simulink model "lte4g"  (R2020b)
settings: Solver=ode45  StartTime=0.0  StopTime=5  RelTol=1e-3  EnableMultiTasking=on
undefined symbols (not defined in the file or in its folder): doppler, Iter, Len, Max, Variance
libraries: commblkintrlv2 x12, dspindex x10, dspobslib x10, commsequence2 x10, commcnvcod2 x8, commchan3 x4, commcrc2 x4, commdigbbndam3 x4, dspxfrm3 x4, commseqgen3 x4, commutil2 x4, opclib x3
settings Model: Creator=Natalia  LastModifiedBy=nitas
settings DataIOCC: LimitDataPoints=on  SaveFormat=Array  SignalLoggingSaveFormat=ModelDataLogs  ReturnWorkspaceOutputs=off
settings OptimizationCC: ExpressionDepthLimit=2147483647  LifeSpan=inf
settings DebuggingCC: UnderspecifiedInitializationDetection=Classic  MergeDetectMultiDrivingBlocksExec=none  SolverPrmCheckMsg=warning  StateNameClashWarn=warning  SFUnexpectedBacktrackingDiag=warning  SFNoUnconditionalDefaultTransitionDiag=warning  SFExecutionAtInitializationDiag=none  ArithmeticOperatorsInVariantConditions=warning
settings HardwareCC: ProdBitPerPointer=32  ProdBitPerSizeT=32  ProdBitPerPtrDiffT=32  ProdLargestAtomicFloat=None  ProdIntDivRoundTo=Undefined  ProdEndianess=Unspecified  ProdWordSize=32  ProdHWDeviceType=32-bit Generic
settings ModelReferenceCC: PropagateSignalLabelsOutOfModel=off
settings SFSimCC: SimUseLocalCustomCode=off  SimParseCustomCode=off  CustomCodeUndefinedFunction=UseInterfaceOnly
settings RTWCC: RTWUseLocalCustomCode=off
settings CodeAppCC: StateflowObjectComments=on
settings GRTTargetCC: TargetLangStandard=C89/C90 (ANSI)  CombineOutputUpdateFcns=off  GRTInterface=on
settings ConfigComp: CovMetricSettings=dw  CovSaveCumulativeToWorkspaceVar=on  CovSaveSingleToWorkspaceVar=on  CovExternalEMLEnable=off

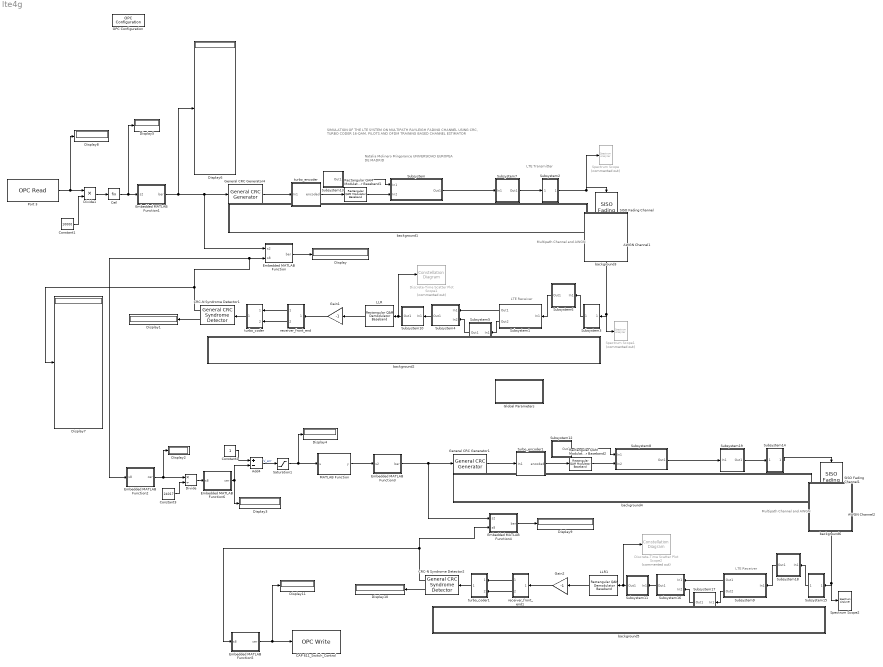
== system lte4g ==
  note: SIMULATION OF THE LTE SYSTEM ON MULTIPATH RAYLEIGH FADING CHANNEL
      | USING CRC, TURBO CODER 16-QAM, PILOTS AND OFDM
      | TRAINING BASED CHANNEL ESTIMATOR
  note: Natalia Molinero Mingorance
      | UNIVERSIDAD EUROPEA DE MADRID
  note: LTE Transmitter
  note: LTE Receiver
  note: Multipath Channel
      | and AWGN
  note: LTE Receiver
  note: Multipath Channel
      | and AWGN
  AWGN Channel1 : commchan3/AWGN Channel  InputProcessing=Columns as channels (frame based)  seed=32965  noiseMode="Signal to noise ratio  (Es/No)"  EbNodB=10  EsNodB=5  SNRdB=0  bitsPerSym=1  Ps=30/(5.5e5*11/15*2.4)*1.08  Tsym=80e-6  variance=1
  AWGN Channel2 : commchan3/AWGN Channel  InputProcessing=Columns as channels (frame based)  seed=32965  noiseMode="Signal to noise ratio  (Es/No)"  EbNodB=10  EsNodB=5  SNRdB=0  bitsPerSym=1  Ps=30/(5.5e5*11/15*2.4)*1.08  Tsym=80e-6  variance=1
  Add4 : Sum  Inputs=+-
  CAP 611_Switch_Control : opclib/OPC Write  serverHost=localhost  serverID=Matrikon.OPC.Simulation.1  itemIDs=Feeder 611.SWT_CAP_611  writeMode=Asynchronous  updateRate=0.01
      settings: SourceProductBaseCode=OT
  CRC-N Syndrome Detector1 : commcrc2/General CRC Syndrome Detector  genPoly=[1 1 0 0 0 0 0 0 0 0 1 0 1 0 0 0 1 0 0 0 0 0 0 0 1]  iniStates=[0]  directMethod=off  reflectInputBytes=off  reflectChecksums=off  finalXOR=0  numChecksums=1
      settings: SourceProductBaseCode=CM
  CRC-N Syndrome Detector2 : commcrc2/General CRC Syndrome Detector  genPoly=[1 1 0 0 0 0 0 0 0 0 1 0 1 0 0 0 1 0 0 0 0 0 0 0 1]  iniStates=[0]  directMethod=off  reflectInputBytes=off  reflectChecksums=off  finalXOR=0  numChecksums=1
      settings: SourceProductBaseCode=CM
  Ceil : Rounding  Operator=fix
  Constant1 : Constant  Value=10000
  Constant2 : Constant
  Constant3 : Constant  Value=24017
  Discrete-Time Scatter Plot Scope1 : ConstellationDiagram  Tag=ScatterPlot  Commented=on
  Discrete-Time Scatter Plot Scope2 : ConstellationDiagram  Tag=ScatterPlot  Commented=on
  Display{,1..11} (12 alike) : Display
  Divide : Product  Inputs=*/
  Divide1 : Product
  Embedded MATLAB Function : MATLAB Function  TreatAsAtomicUnit=on
  Embedded MATLAB Function1 : MATLAB Function  TreatAsAtomicUnit=on
  Embedded MATLAB Function2 : MATLAB Function  TreatAsAtomicUnit=on
  Embedded MATLAB Function3 : MATLAB Function  TreatAsAtomicUnit=on
  Embedded MATLAB Function4 : MATLAB Function  TreatAsAtomicUnit=on
  Embedded MATLAB Function5 : MATLAB Function  TreatAsAtomicUnit=on
  Embedded MATLAB Function6 : MATLAB Function  TreatAsAtomicUnit=on
  Gain1 : Gain  Gain=-1  SaturateOnIntegerOverflow=on  OutDataTypeStr=Inherit: Same as input  ParamDataTypeStr=Inherit: Same as input
  Gain2 : Gain  Gain=-1  SaturateOnIntegerOverflow=on  OutDataTypeStr=Inherit: Same as input  ParamDataTypeStr=Inherit: Same as input
  General CRC Generator1 : commcrc2/General CRC Generator  genPoly=[24,23,6,5,1,0]  iniStates=[0]  directMethod=off  reflectInputBytes=off  reflectChecksums=off  finalXOR=0  numChecksums=1
      settings: SourceProductBaseCode=CM
  General CRC Generator4 : commcrc2/General CRC Generator  genPoly=[24,23,6,5,1,0]  iniStates=[0]  directMethod=off  reflectInputBytes=off  reflectChecksums=off  finalXOR=0  numChecksums=1
      settings: SourceProductBaseCode=CM
  Global Parameters : Subsystem  mask(Global Parameters){EbNodB=11, Len=44, Iter=5, Seed=54123}
      mask prompts: EbNodB "Eb/No in dB:"; Len "Block size:"; Iter "Number of iterations:"
      mask help: Load global parameters in MATLAB workspace.
      mask init:
      | turbo_code_punc_setup;
      mask Callback EbNodB: turbo_code_setup;
      mask Callback Len: turbo_code_setup
      mask Callback Iter: turbo_code_setup;
      mask Callback Seed: turbo_code_setup;
      mask Display: disp(['Eb/No ' num2str(EbNodB,'%3.1f') 'dB'  sprintf('\n') 'Block size   ' num2str(Len,'%7.0f')  sprintf('\n') 'Iterations   ' num2str(Iter,'%3.0f')   sprintf('\n') 'Seed   ' num2str(Seed,'%7.0f')])
  LLR : commdigbbndam3/Rectangular QAM Demodulator Baseband  M=16  OutType=Bit  DecType=Log-likelihood ratio  VarSource=Dialog  Variance=Variance  Dec=Gray  Mapping=[0:15]  PowType=Average Power  MinDist=2  AvgPow=0.5  PeakPow=1  Ph=0  outDtype1=double  outDtype2=double  derotateFactorWordLen=16  derotateFactorDataTypeStr=Inherit: Same word length as input  derotateFactorLastDataTypeStr=Inherit: Same word length as input  denormFactorWordLen=16  denormFactorDataTypeStr=Inherit: Same word length as input  denormFactorLastDataTypeStr=Inherit: Same word length as input  prodOutWordLen=32  prodOutOverflowMode=Wrap  prodOutRoundingMode=Floor  prodOutOvFlMode=off  prodOutOvFlModeLastStrValue=off  sumWordLen=32
  LLR1 : commdigbbndam3/Rectangular QAM Demodulator Baseband  M=16  OutType=Bit  DecType=Log-likelihood ratio  VarSource=Dialog  Variance=Variance  Dec=Gray  Mapping=[0:15]  PowType=Average Power  MinDist=2  AvgPow=0.5  PeakPow=1  Ph=0  outDtype1=double  outDtype2=double  derotateFactorWordLen=16  derotateFactorDataTypeStr=Inherit: Same word length as input  derotateFactorLastDataTypeStr=Inherit: Same word length as input  denormFactorWordLen=16  denormFactorDataTypeStr=Inherit: Same word length as input  denormFactorLastDataTypeStr=Inherit: Same word length as input  prodOutWordLen=32  prodOutOverflowMode=Wrap  prodOutRoundingMode=Floor  prodOutOvFlMode=off  prodOutOvFlModeLastStrValue=off  sumWordLen=32
  MATLAB Function : MATLAB Function  TreatAsAtomicUnit=on
  OPC Configuration : opclib/OPC Configuration  opcServers=localhost/Matrikon.OPC.Simulation.1/10  errMissingItems=Warn  errReadWrite=Warn  errShutdown=Warn  errRTViolation=Warn  rtEnable=off  speedup=1  showLatency=off  beingUsed=on
      settings: SourceProductBaseCode=OT
  Port 3 : opclib/OPC Read  serverHost=localhost  serverID=Matrikon.OPC.Simulation.1  itemIDs=Feeder 611.LOAD_611_V_RES  readMode=Asynchronous (device)  dataType=double  updateRate=0.01  showQual=off  showTS=off  tsMode=Seconds since start
      settings: SourceProductBaseCode=OT
  Rectangular QAM Modulator Baseband1 : commdigbbndam3/Rectangular QAM Modulator Baseband  M=16  InType=Bit  Enc=Gray  Mapping=[0:15]  PowType=Average Power  MinDist=2  AvgPow=0.5  PeakPow=1  Ph=0  outDtype=double  outWordLen=16  outUDDataType=sfix(16)  outFracLenMode=Best precision  outFracLen=15  outDataTypeStr=double  outLastDataTypeStr=double
  Rectangular QAM Modulator Baseband2 : commdigbbndam3/Rectangular QAM Modulator Baseband  M=16  InType=Bit  Enc=Gray  Mapping=[0:15]  PowType=Average Power  MinDist=2  AvgPow=0.5  PeakPow=1  Ph=0  outDtype=double  outWordLen=16  outUDDataType=sfix(16)  outFracLenMode=Best precision  outFracLen=15  outDataTypeStr=double  outLastDataTypeStr=double
  SISO Fading Channel : commchan3/SISO Fading Channel  InheritSampleRate=on  SampleRate=1  PathDelays=0  AveragePathGains=0  NormalizePathGains=on  FadingDistribution=Rayleigh  KFactor=3  DirectPathDopplerShift=0  DirectPathInitialPhase=0  MaximumDopplerShift=0.001  DopplerSpectrum=doppler('Jakes')  RandomStream=mt19937ar with seed  Seed=73  PathGainsOutputPort=off  ChannelFilterDelayOutputPort=off  SimulateUsing=Interpreted execution  Visualization=Off  PathsForDopplerDisplay=1  SamplesToDisplay=25%
  SISO Fading Channel1 : commchan3/SISO Fading Channel  InheritSampleRate=on  SampleRate=1  PathDelays=0  AveragePathGains=0  NormalizePathGains=on  FadingDistribution=Rayleigh  KFactor=3  DirectPathDopplerShift=0  DirectPathInitialPhase=0  MaximumDopplerShift=0.001  DopplerSpectrum=doppler('Jakes')  RandomStream=mt19937ar with seed  Seed=73  PathGainsOutputPort=off  ChannelFilterDelayOutputPort=off  SimulateUsing=Interpreted execution  Visualization=Off  PathsForDopplerDisplay=1  SamplesToDisplay=25%
  Saturation1 : Saturate  UpperLimit=0.05  LowerLimit=-0.05
  Spectrum Scope : SpectrumAnalyzer  Commented=on
  Spectrum Scope1 : SpectrumAnalyzer  Commented=on
  Spectrum Scope2 : SpectrumAnalyzer
  Subsystem : Subsystem
      mask Display: disp('OFDM Baseband\nModulator\ndan\nAdd Cyclic Prefix')
  Subsystem1 : Subsystem
      mask Display: disp('OFDM Baseband\nDemodulator\ndan \nRemove Cyclic prefix')
  Subsystem10 : Subsystem
      mask Display: disp('Remove\nZero')
  Subsystem11 : Subsystem
      mask Display: disp('Remove\nZero')
  Subsystem12 : Subsystem
      mask Display: disp('Training')
  Subsystem13 : Subsystem
      mask Display: disp('Training')
  Subsystem14 : Subsystem
      mask Display: disp('P/S')
  Subsystem15 : Subsystem
      mask Display: disp('S/P')
  Subsystem16 : Subsystem
      mask Display: disp('Channel\nCompensation')
  Subsystem17 : Subsystem
      mask Display: disp('Channel\nEstimator')
  Subsystem18 : Subsystem
      mask Display: disp('Training\nSeparation')
  Subsystem19 : Subsystem
      mask Display: disp('Training\nInsertion')
  Subsystem2 : Subsystem
      mask Display: disp('P/S')
  Subsystem3 : Subsystem
      mask Display: disp('S/P')
  Subsystem4 : Subsystem
      mask Display: disp('Channel\nCompensation')
  Subsystem5 : Subsystem
      mask Display: disp('Channel\nEstimator')
  Subsystem6 : Subsystem
      mask Display: disp('Training\nSeparation')
  Subsystem7 : Subsystem
      mask Display: disp('Training\nInsertion')
  Subsystem8 : Subsystem
      mask Display: disp('OFDM Baseband\nModulator\ndan\nAdd Cyclic Prefix')
  Subsystem9 : Subsystem
      mask Display: disp('OFDM Baseband\nDemodulator\ndan \nRemove Cyclic prefix')
  background1 : Subsystem
      mask Display: disp('')
  background2 : Subsystem
      mask Display: disp('')
  background3 : Subsystem
      mask Display: disp('')
  background4 : Subsystem
      mask Display: disp('')
  background5 : Subsystem
      mask Display: disp('')
  background6 : Subsystem
      mask Display: disp('')
  receiver_front_end : Subsystem
  receiver_front_end1 : Subsystem
  turbo_coder : Subsystem
  turbo_coder1 : Subsystem
  turbo_encoder : Subsystem
  turbo_encoder1 : Subsystem
  wires:
  receiver_front_end/1(Out1) -> turbo_coder/1(In1)
  receiver_front_end/2(Out2) -> turbo_coder/2(In2)
  turbo_encoder/1(encoded) -> Rectangular QAM Modulator Baseband1/1
  LLR/1 -> Gain1/1
  Gain1/1 -> receiver_front_end/1(In1)
  Subsystem13/1(Out1) -> Subsystem/1(In1)
  Subsystem/1(Out1) -> Subsystem7/1(In1)
  Subsystem7/1(Out1) -> Subsystem2/1(In1)
  Rectangular QAM Modulator Baseband1/1 -> Subsystem/2(In2)
  Subsystem1/1(Out1) -> Subsystem4/1(In1)
  Subsystem1/2(Out2) -> Subsystem5/1(In1)
  Subsystem5/1(Out1) -> Subsystem4/2(In2)
  Subsystem4/1(Out1) -> Subsystem10/1(In1)
  Subsystem6/1(Out1) -> Subsystem1/1(In1)
  Subsystem3/1(Out1) -> Subsystem6/1(In1)
  Subsystem10/1(Out1) -> LLR/1, Discrete-Time Scatter Plot Scope1/1
  SISO Fading Channel/1 -> AWGN Channel1/1
  AWGN Channel1/1 -> Subsystem3/1(In1), Spectrum Scope1/1
  Subsystem2/1(Out1) -> SISO Fading Channel/1, Spectrum Scope/1
  General CRC Generator4/1 -> turbo_encoder/1(In1)
  turbo_coder/1(Out1) -> CRC-N Syndrome Detector1/1
  Embedded MATLAB Function/1(ber) -> Display/1
  CRC-N Syndrome Detector1/2 -> Display1/1
  Ceil/1 -> Embedded MATLAB Function1/1(s2), Display5/1
  CRC-N Syndrome Detector1/1 -> Embedded MATLAB Function2/1(s8), Embedded MATLAB Function/2(s8), Display7/1
  Saturation1/1 -> Display4/1, MATLAB Function/1(u)
  Add4/1 -> Saturation1/1  "V_err"
  Constant2/1 -> Add4/1
  Embedded MATLAB Function2/1(cer) -> Divide/1, Display2/1
  Port 3/1 -> Display8/1, Divide1/1
  Divide1/1 -> Ceil/1
  Constant1/1 -> Divide1/2
  Embedded MATLAB Function1/1(ber) -> Display6/1, Embedded MATLAB Function/1(s2), General CRC Generator4/1
  MATLAB Function/1(y) -> Embedded MATLAB Function3/1(s2)
  Embedded MATLAB Function3/1(ber) -> Embedded MATLAB Function4/1(s2), General CRC Generator1/1
  Subsystem12/1(Out1) -> Subsystem8/1(In1)
  CRC-N Syndrome Detector2/2 -> Display10/1
  Subsystem9/2(Out2) -> Subsystem17/1(In1)
  Subsystem9/1(Out1) -> Subsystem16/1(In1)
  AWGN Channel2/1 -> Subsystem15/1(In1), Spectrum Scope2/1
  turbo_coder1/1(Out1) -> CRC-N Syndrome Detector2/1
  receiver_front_end1/1(Out1) -> turbo_coder1/1(In1)
  Subsystem14/1(Out1) -> SISO Fading Channel1/1
  LLR1/1 -> Gain2/1
  Subsystem8/1(Out1) -> Subsystem19/1(In1)
  Subsystem11/1(Out1) -> LLR1/1, Discrete-Time Scatter Plot Scope2/1
  Subsystem15/1(Out1) -> Subsystem18/1(In1)
  Rectangular QAM Modulator Baseband2/1 -> Subsystem8/2(In2)
  CRC-N Syndrome Detector2/1 -> Embedded MATLAB Function5/1(s8), Embedded MATLAB Function4/2(s8)
  Embedded MATLAB Function4/1(ber) -> Display9/1
  Subsystem16/1(Out1) -> Subsystem11/1(In1)
  General CRC Generator1/1 -> turbo_encoder1/1(In1)
  SISO Fading Channel1/1 -> AWGN Channel2/1
  Subsystem18/1(Out1) -> Subsystem9/1(In1)
  receiver_front_end1/2(Out2) -> turbo_coder1/2(In2)
  Gain2/1 -> receiver_front_end1/1(In1)
  Subsystem17/1(Out1) -> Subsystem16/2(In2)
  Subsystem19/1(Out1) -> Subsystem14/1(In1)
  turbo_encoder1/1(encoded) -> Rectangular QAM Modulator Baseband2/1
  Embedded MATLAB Function5/1(cer) -> Display11/1, CAP 611_Switch_Control/1
  Constant3/1 -> Divide/2
  Divide/1 -> Embedded MATLAB Function6/1(s8)
  Embedded MATLAB Function6/1(cer) -> Display3/1, Add4/2

== system lte4g/Global Parameters ==

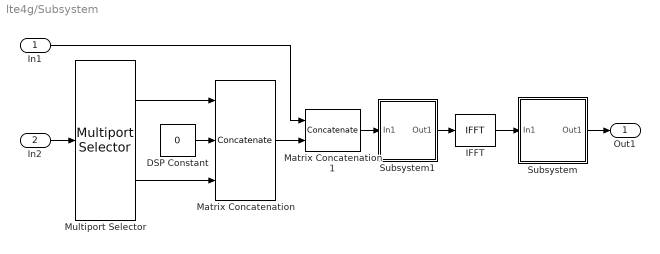
== system lte4g/Subsystem ==
  In1 : Inport
  In2 : Inport  Port=2
  DSP Constant : Constant  Value=0  VectorParams1D=off  FramePeriod=16e-5/2
      settings: SamplingMode=Frame based
  IFFT : dspxfrm3/IFFT  FFTImplementation=Auto  CompMethod=Table lookup  TableOpt=HYBRID  TableOptActive=Speed  BitRevOrder=off  cs_in=off  Normalize=on  InheritFFTLength=on  FFTLength=64  WrapInput=on  mode=Real  outSamplingMode=Frame based  roundingMode=Floor  overflowMode=off  firstCoeffDataTypeStr=Inherit: Same word length as input  firstCoeffLastDataTypeStr=Inherit: Same word length as input  outputMin=[]  outputMax=[]
  Matrix Concatenation : Concatenate  NumInputs=3  Mode=Multidimensional array
  Matrix Concatenation1 : Concatenate  Mode=Multidimensional array  ConcatenateDimension=2
  Multiport Selector : dspindex/Multiport Selector  rowsOrCols=Rows  idxCellArray={1:11,12:22}  idxErrMode=Clip Index
  Subsystem : Subsystem
      mask Display: disp('Add\nCyclic Prefix')
  Subsystem1 : Subsystem
      mask Display: disp('Zero Pad')
  Out1 : Outport
  wires:
  IFFT/1 -> Subsystem/1(In1)
  Multiport Selector/1 -> Matrix Concatenation/1
  Multiport Selector/2 -> Matrix Concatenation/3
  DSP Constant/1 -> Matrix Concatenation/2
  Subsystem1/1(Out1) -> IFFT/1
  Subsystem/1(Out1) -> Out1/1
  In2/1 -> Multiport Selector/1
  Matrix Concatenation1/1 -> Subsystem1/1(In1)
  Matrix Concatenation/1 -> Matrix Concatenation1/2
  In1/1 -> Matrix Concatenation1/1

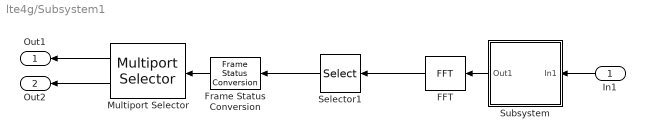
== system lte4g/Subsystem1 ==
  In1 : Inport
  FFT : dspxfrm3/FFT  FFTImplementation=Auto  CompMethod=Table lookup  TableOpt=NEW  TableOptActive=Speed  BitRevOrder=off  Normalize=on  InheritFFTLength=on  FFTLength=64  WrapInput=on  roundingMode=Floor  overflowMode=off  firstCoeffDataTypeStr=Inherit: Same word length as input  firstCoeffLastDataTypeStr=Inherit: Same word length as input  outputMin=[]  outputMax=[]
  Frame Status Conversion : dspobslib/Frame Status Conversion  growRefPort=off  outframe=Frame-based
      settings: SourceProductBaseCode=DS
  Multiport Selector : dspindex/Multiport Selector  rowsOrCols=Columns  idxCellArray={1,2}  idxErrMode=Clip Index
  Selector1 : Selector  NumberOfDimensions=2  InputPortWidth=64  IndexOptions=Index vector (dialog),Select all  Indices=[54:64,1:12],-1  OutputSizes=1
  Subsystem : Subsystem
      mask Display: disp('Remove\nCyclic Prefix')
  Out1 : Outport
  Out2 : Outport  Port=2
  wires:
  FFT/1 -> Selector1/1
  Selector1/1 -> Frame Status Conversion/1
  Subsystem/1(Out1) -> FFT/1
  In1/1 -> Subsystem/1(In1)
  Frame Status Conversion/1 -> Multiport Selector/1
  Multiport Selector/1 -> Out1/1
  Multiport Selector/2 -> Out2/1

== system lte4g/Subsystem10 ==
  In1 : Inport
  Selector2 : Selector  NumberOfDimensions=2  InputPortWidth=31  IndexOptions=Index vector (dialog),Select all  Indices=[1:11,13:23],-1  OutputSizes=1
  Out1 : Outport
  tag scope: konstelasi_stl1=global
  wires:
  Selector2/1 -> Out1/1, [konstelasi_stl1]
  In1/1 -> Selector2/1

== system lte4g/Subsystem11 ==
  In1 : Inport
  Selector2 : Selector  NumberOfDimensions=2  InputPortWidth=31  IndexOptions=Index vector (dialog),Select all  Indices=[1:11,13:23],-1  OutputSizes=1
  Out1 : Outport
  tag scope: konstelasi_stl=global
  wires:
  Selector2/1 -> Out1/1, [konstelasi_stl]
  In1/1 -> Selector2/1

== system lte4g/Subsystem12 ==
  PN Sequence Generator : commseqgen3/PN Sequence Generator  poly=[1 0 0 0 0 1 1]  ini_sta=[0 0 0 0 0 1]  outBitMaskSource=Dialog parameter  shift=0  outVarSiz=off  maxOutSizeMode=Dialog parameter  maxOutSize=[10 1]  Ts=16e-5/2/23  sampPerFrame=23  reset=off  bitPackedOutputs=off  outDataType=double  numPackedBits=8  bitPackDataSigned=off  bitPackedOutDType=double
  Unipolar to Bipolar Converter : commutil2/Unipolar to Bipolar Converter  M=2  polarity=Positive  dataType=Inherit via internal rule
  Out1 : Outport
  wires:
  PN Sequence Generator/1 -> Unipolar to Bipolar Converter/1
  Unipolar to Bipolar Converter/1 -> Out1/1

== system lte4g/Subsystem13 ==
  PN Sequence Generator : commseqgen3/PN Sequence Generator  poly=[1 0 0 0 0 1 1]  ini_sta=[0 0 0 0 0 1]  outBitMaskSource=Dialog parameter  shift=0  outVarSiz=off  maxOutSizeMode=Dialog parameter  maxOutSize=[10 1]  Ts=16e-5/2/23  sampPerFrame=23  reset=off  bitPackedOutputs=off  outDataType=double  numPackedBits=8  bitPackDataSigned=off  bitPackedOutDType=double
  Unipolar to Bipolar Converter : commutil2/Unipolar to Bipolar Converter  M=2  polarity=Positive  dataType=Inherit via internal rule
  Out1 : Outport
  wires:
  PN Sequence Generator/1 -> Unipolar to Bipolar Converter/1
  Unipolar to Bipolar Converter/1 -> Out1/1

== system lte4g/Subsystem14 ==
  In1 : Inport
  Unbuffer3 : Unbuffer
  Out1 : Outport
  wires:
  In1/1 -> Unbuffer3/1
  Unbuffer3/1 -> Out1/1

== system lte4g/Subsystem15 ==
  In1 : Inport
  Buffer : Buffer  N=180
  Complex to Real-Imag : ComplexToRealImag
  Out1 : Outport
  tag scope: im_rx=global, real_rx=global, spektrum_terima=global
  wires:
  In1/1 -> Buffer/1, [spektrum_terima], Complex to Real-Imag/1
  Buffer/1 -> Out1/1
  Complex to Real-Imag/1 -> [real_rx]
  Complex to Real-Imag/2 -> [im_rx]

== system lte4g/Subsystem16 ==
  In1 : Inport
  In2 : Inport  Port=2
  Frame Status Conversion5 : dspobslib/Frame Status Conversion  growRefPort=off  outframe=Frame-based
      settings: SourceProductBaseCode=DS
  Product : Product  SaturateOnIntegerOverflow=on  OutDataTypeStr=Inherit: Same as first input
  Out1 : Outport
  wires:
  Product/1 -> Frame Status Conversion5/1
  Frame Status Conversion5/1 -> Out1/1
  In2/1 -> Product/1
  In1/1 -> Product/2

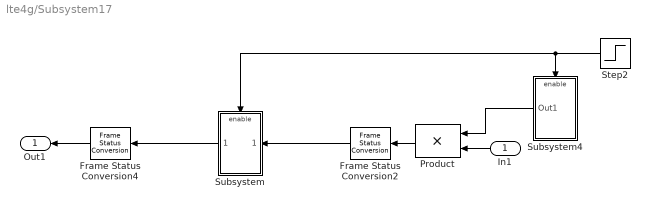
== system lte4g/Subsystem17 ==
  In1 : Inport
  Frame Status Conversion2 : dspobslib/Frame Status Conversion  growRefPort=off  outframe=Frame-based
      settings: SourceProductBaseCode=DS
  Frame Status Conversion4 : dspobslib/Frame Status Conversion  growRefPort=off  outframe=Frame-based
      settings: SourceProductBaseCode=DS
  Product : Product  SaturateOnIntegerOverflow=on  OutDataTypeStr=Inherit: Same as first input
  Step2 : Step  Time=16e-5/2  SampleTime=16e-5/2
  Subsystem : Subsystem
  Subsystem4 : Subsystem  TreatAsAtomicUnit=on
  Out1 : Outport
  wires:
  Step2/1 -> Subsystem4/Enable, Subsystem/Enable
  Subsystem4/1(Out1) -> Product/1
  Product/1 -> Frame Status Conversion2/1
  Frame Status Conversion2/1 -> Subsystem/1(In1)
  Frame Status Conversion4/1 -> Out1/1
  In1/1 -> Product/2
  Subsystem/1(Out1) -> Frame Status Conversion4/1

== system lte4g/Subsystem18 ==
  In1 : Inport
  Matrix Concatenation1 : Concatenate  Mode=Multidimensional array  ConcatenateDimension=2
  Multiport Selector1 : dspindex/Multiport Selector  rowsOrCols=Rows  idxCellArray={91:180,1:90}  idxErrMode=Clip Index
  Out1 : Outport
  wires:
  Multiport Selector1/2 -> Matrix Concatenation1/2
  Multiport Selector1/1 -> Matrix Concatenation1/1
  In1/1 -> Multiport Selector1/1
  Matrix Concatenation1/1 -> Out1/1

== system lte4g/Subsystem19 ==
  In1 : Inport
  Matrix Concatenation : Concatenate  Mode=Multidimensional array
  Multiport Selector : dspindex/Multiport Selector  rowsOrCols=Columns  idxCellArray={1,2}  idxErrMode=Clip Index
  Out1 : Outport
  wires:
  Multiport Selector/1 -> Matrix Concatenation/1
  Multiport Selector/2 -> Matrix Concatenation/2
  In1/1 -> Multiport Selector/1
  Matrix Concatenation/1 -> Out1/1

== system lte4g/Subsystem2 ==
  In1 : Inport
  Unbuffer3 : Unbuffer
  Out1 : Outport
  wires:
  In1/1 -> Unbuffer3/1
  Unbuffer3/1 -> Out1/1

== system lte4g/Subsystem3 ==
  In1 : Inport
  Buffer : Buffer  N=180
  Complex to Real-Imag : ComplexToRealImag
  Out1 : Outport
  tag scope: im_rx1=global, real_rx1=global, spektrum_terima1=global
  wires:
  In1/1 -> Buffer/1, [spektrum_terima1], Complex to Real-Imag/1
  Buffer/1 -> Out1/1
  Complex to Real-Imag/1 -> [real_rx1]
  Complex to Real-Imag/2 -> [im_rx1]

== system lte4g/Subsystem4 ==
  In1 : Inport
  In2 : Inport  Port=2
  Frame Status Conversion5 : dspobslib/Frame Status Conversion  growRefPort=off  outframe=Frame-based
      settings: SourceProductBaseCode=DS
  Product : Product  SaturateOnIntegerOverflow=on  OutDataTypeStr=Inherit: Same as first input
  Out1 : Outport
  wires:
  Product/1 -> Frame Status Conversion5/1
  Frame Status Conversion5/1 -> Out1/1
  In2/1 -> Product/1
  In1/1 -> Product/2

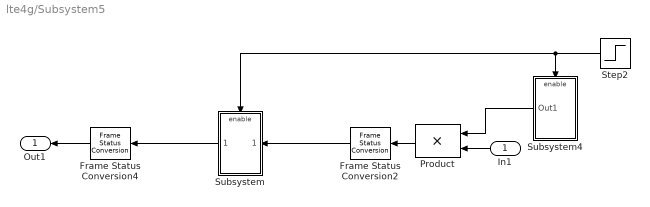
== system lte4g/Subsystem5 ==
  In1 : Inport
  Frame Status Conversion2 : dspobslib/Frame Status Conversion  growRefPort=off  outframe=Frame-based
      settings: SourceProductBaseCode=DS
  Frame Status Conversion4 : dspobslib/Frame Status Conversion  growRefPort=off  outframe=Frame-based
      settings: SourceProductBaseCode=DS
  Product : Product  SaturateOnIntegerOverflow=on  OutDataTypeStr=Inherit: Same as first input
  Step2 : Step  Time=16e-5/2  SampleTime=16e-5/2
  Subsystem : Subsystem
  Subsystem4 : Subsystem  TreatAsAtomicUnit=on
  Out1 : Outport
  wires:
  Step2/1 -> Subsystem4/Enable, Subsystem/Enable
  Subsystem4/1(Out1) -> Product/1
  Product/1 -> Frame Status Conversion2/1
  Frame Status Conversion2/1 -> Subsystem/1(In1)
  Frame Status Conversion4/1 -> Out1/1
  In1/1 -> Product/2
  Subsystem/1(Out1) -> Frame Status Conversion4/1

== system lte4g/Subsystem6 ==
  In1 : Inport
  Matrix Concatenation1 : Concatenate  Mode=Multidimensional array  ConcatenateDimension=2
  Multiport Selector1 : dspindex/Multiport Selector  rowsOrCols=Rows  idxCellArray={91:180,1:90}  idxErrMode=Clip Index
  Out1 : Outport
  wires:
  Multiport Selector1/2 -> Matrix Concatenation1/2
  Multiport Selector1/1 -> Matrix Concatenation1/1
  In1/1 -> Multiport Selector1/1
  Matrix Concatenation1/1 -> Out1/1

== system lte4g/Subsystem7 ==
  In1 : Inport
  Matrix Concatenation : Concatenate  Mode=Multidimensional array
  Multiport Selector : dspindex/Multiport Selector  rowsOrCols=Columns  idxCellArray={1,2}  idxErrMode=Clip Index
  Out1 : Outport
  wires:
  Multiport Selector/1 -> Matrix Concatenation/1
  Multiport Selector/2 -> Matrix Concatenation/2
  In1/1 -> Multiport Selector/1
  Matrix Concatenation/1 -> Out1/1

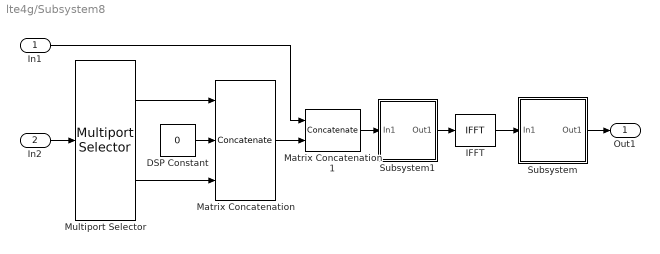
== system lte4g/Subsystem8 ==
  In1 : Inport
  In2 : Inport  Port=2
  DSP Constant : Constant  Value=0  VectorParams1D=off  FramePeriod=16e-5/2
      settings: SamplingMode=Frame based
  IFFT : dspxfrm3/IFFT  FFTImplementation=Auto  CompMethod=Table lookup  TableOpt=HYBRID  TableOptActive=Speed  BitRevOrder=off  cs_in=off  Normalize=on  InheritFFTLength=on  FFTLength=64  WrapInput=on  mode=Real  outSamplingMode=Frame based  roundingMode=Floor  overflowMode=off  firstCoeffDataTypeStr=Inherit: Same word length as input  firstCoeffLastDataTypeStr=Inherit: Same word length as input  outputMin=[]  outputMax=[]
  Matrix Concatenation : Concatenate  NumInputs=3  Mode=Multidimensional array
  Matrix Concatenation1 : Concatenate  Mode=Multidimensional array  ConcatenateDimension=2
  Multiport Selector : dspindex/Multiport Selector  rowsOrCols=Rows  idxCellArray={1:11,12:22}  idxErrMode=Clip Index
  Subsystem : Subsystem
      mask Display: disp('Add\nCyclic Prefix')
  Subsystem1 : Subsystem
      mask Display: disp('Zero Pad')
  Out1 : Outport
  wires:
  IFFT/1 -> Subsystem/1(In1)
  Multiport Selector/1 -> Matrix Concatenation/1
  Multiport Selector/2 -> Matrix Concatenation/3
  DSP Constant/1 -> Matrix Concatenation/2
  Subsystem1/1(Out1) -> IFFT/1
  Subsystem/1(Out1) -> Out1/1
  In2/1 -> Multiport Selector/1
  Matrix Concatenation1/1 -> Subsystem1/1(In1)
  Matrix Concatenation/1 -> Matrix Concatenation1/2
  In1/1 -> Matrix Concatenation1/1

== system lte4g/Subsystem9 ==
  In1 : Inport
  FFT : dspxfrm3/FFT  FFTImplementation=Auto  CompMethod=Table lookup  TableOpt=NEW  TableOptActive=Speed  BitRevOrder=off  Normalize=on  InheritFFTLength=on  FFTLength=64  WrapInput=on  roundingMode=Floor  overflowMode=off  firstCoeffDataTypeStr=Inherit: Same word length as input  firstCoeffLastDataTypeStr=Inherit: Same word length as input  outputMin=[]  outputMax=[]
  Frame Status Conversion : dspobslib/Frame Status Conversion  growRefPort=off  outframe=Frame-based
      settings: SourceProductBaseCode=DS
  Multiport Selector : dspindex/Multiport Selector  rowsOrCols=Columns  idxCellArray={1,2}  idxErrMode=Clip Index
  Selector1 : Selector  NumberOfDimensions=2  InputPortWidth=64  IndexOptions=Index vector (dialog),Select all  Indices=[54:64,1:12],-1  OutputSizes=1
  Subsystem : Subsystem
      mask Display: disp('Remove\nCyclic Prefix')
  Out1 : Outport
  Out2 : Outport  Port=2
  wires:
  FFT/1 -> Selector1/1
  Selector1/1 -> Frame Status Conversion/1
  Subsystem/1(Out1) -> FFT/1
  In1/1 -> Subsystem/1(In1)
  Frame Status Conversion/1 -> Multiport Selector/1
  Multiport Selector/1 -> Out1/1
  Multiport Selector/2 -> Out2/1

== system lte4g/background1 ==

== system lte4g/background2 ==

== system lte4g/background3 ==

== system lte4g/background4 ==

== system lte4g/background5 ==

== system lte4g/background6 ==

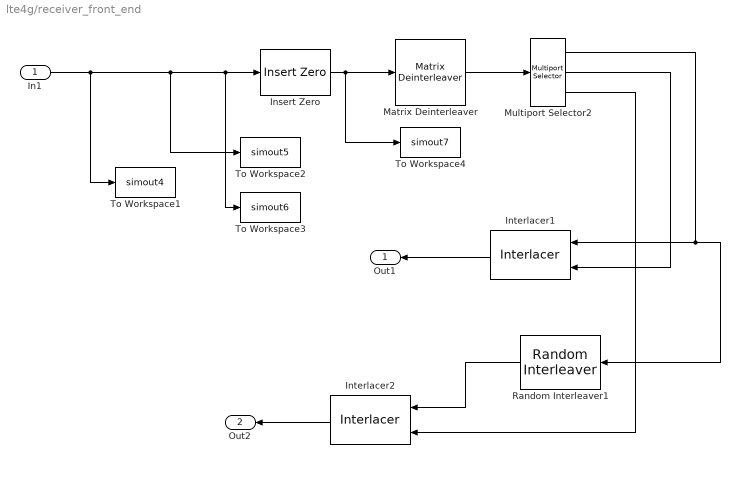
== system lte4g/receiver_front_end ==
  In1 : Inport
  Insert Zero : commobslib/Insert Zero  insertZeroVector=[1 1 0 1 0 1].'
      settings: SourceProductBaseCode=CM
  Interlacer1 : commsequence2/Interlacer
      settings: SourceProductBaseCode=CM
  Interlacer2 : commsequence2/Interlacer
      settings: SourceProductBaseCode=CM
  Matrix Deinterleaver : commblkintrlv2/Matrix Deinterleaver  Nrows=3  Ncols=44
      settings: SourceProductBaseCode=CM
  Multiport Selector2 : dspindex/Multiport Selector  rowsOrCols=Rows  idxCellArray={1:Len, Len+1:2*Len, 2*Len+1:3*Len}  idxErrMode=Clip Index
  Random Interleaver1 : commblkintrlv2/Random Interleaver  N=Len  seed=Seed
      settings: SourceProductBaseCode=CM
  To Workspace1 : ToWorkspace  VariableName=simout4  SampleTime=-1
  To Workspace2 : ToWorkspace  VariableName=simout5  SampleTime=-1
  To Workspace3 : ToWorkspace  VariableName=simout6  SampleTime=-1
  To Workspace4 : ToWorkspace  VariableName=simout7  SampleTime=-1
  Out1 : Outport
  Out2 : Outport  Port=2
  wires:
  Multiport Selector2/1 -> Interlacer1/1, Random Interleaver1/1
  Multiport Selector2/2 -> Interlacer1/2
  Random Interleaver1/1 -> Interlacer2/1
  Multiport Selector2/3 -> Interlacer2/2
  In1/1 -> To Workspace1/1, To Workspace2/1, Insert Zero/1, To Workspace3/1
  Interlacer1/1 -> Out1/1
  Interlacer2/1 -> Out2/1
  Matrix Deinterleaver/1 -> Multiport Selector2/1
  Insert Zero/1 -> Matrix Deinterleaver/1, To Workspace4/1

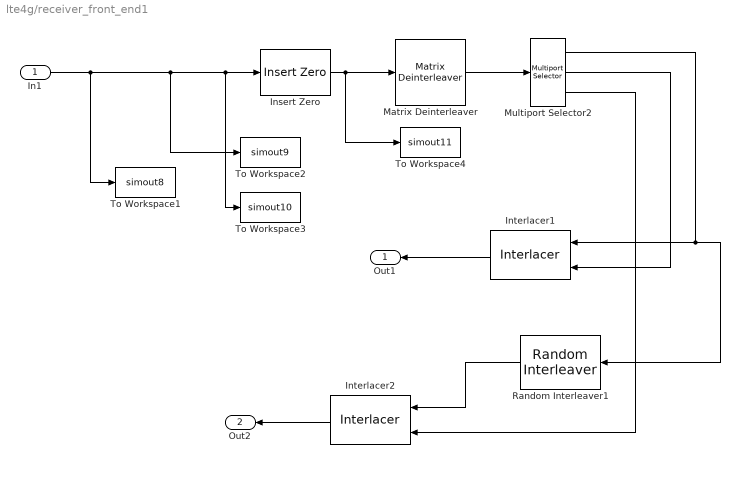
== system lte4g/receiver_front_end1 ==
  In1 : Inport
  Insert Zero : commobslib/Insert Zero  insertZeroVector=[1 1 0 1 0 1].'
      settings: SourceProductBaseCode=CM
  Interlacer1 : commsequence2/Interlacer
      settings: SourceProductBaseCode=CM
  Interlacer2 : commsequence2/Interlacer
      settings: SourceProductBaseCode=CM
  Matrix Deinterleaver : commblkintrlv2/Matrix Deinterleaver  Nrows=3  Ncols=44
      settings: SourceProductBaseCode=CM
  Multiport Selector2 : dspindex/Multiport Selector  rowsOrCols=Rows  idxCellArray={1:Len, Len+1:2*Len, 2*Len+1:3*Len}  idxErrMode=Clip Index
  Random Interleaver1 : commblkintrlv2/Random Interleaver  N=Len  seed=Seed
      settings: SourceProductBaseCode=CM
  To Workspace1 : ToWorkspace  VariableName=simout8  SampleTime=-1
  To Workspace2 : ToWorkspace  VariableName=simout9  SampleTime=-1
  To Workspace3 : ToWorkspace  VariableName=simout10  SampleTime=-1
  To Workspace4 : ToWorkspace  VariableName=simout11  SampleTime=-1
  Out1 : Outport
  Out2 : Outport  Port=2
  wires:
  Multiport Selector2/1 -> Interlacer1/1, Random Interleaver1/1
  Multiport Selector2/2 -> Interlacer1/2
  Random Interleaver1/1 -> Interlacer2/1
  Multiport Selector2/3 -> Interlacer2/2
  In1/1 -> To Workspace1/1, To Workspace2/1, Insert Zero/1, To Workspace3/1
  Interlacer1/1 -> Out1/1
  Interlacer2/1 -> Out2/1
  Matrix Deinterleaver/1 -> Multiport Selector2/1
  Insert Zero/1 -> Matrix Deinterleaver/1, To Workspace4/1

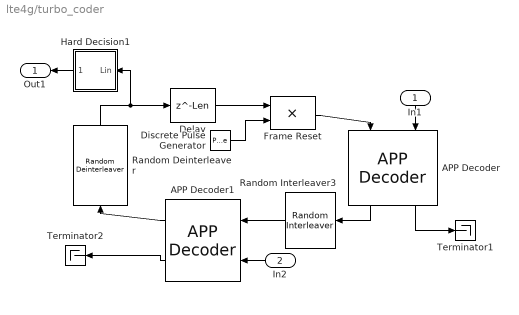
== system lte4g/turbo_coder ==
  In1 : Inport
  In2 : Inport  Port=2
  APP Decoder : commcnvcod2/APP Decoder  trellis=trellis  termMethod=Truncated  algorithm=Max*  maxStarNumScaleBits=3  disableLcOut=off
      settings: SourceProductBaseCode=CM
  APP Decoder1 : commcnvcod2/APP Decoder  trellis=trellis  termMethod=Truncated  algorithm=Max*  maxStarNumScaleBits=3  disableLcOut=off
      settings: SourceProductBaseCode=CM
  Delay : Delay  DelayLength=Len  InitialCondition=0  InputProcessing=Columns as channels (frame based)
  Discrete Pulse Generator : DiscretePulseGenerator  Period=Iter  PulseWidth=Iter-1  PhaseDelay=1
  Frame Reset : Product  InputSameDT=on  SaturateOnIntegerOverflow=on  OutDataTypeStr=Inherit: Same as first input
  Hard Decision1 : Subsystem  mask(Hard Decision){}
      mask help: Likelihood to binary transformation.
  Random Deinterleaver : commblkintrlv2/Random Deinterleaver  N=Len  seed=Seed
      settings: SourceProductBaseCode=CM
  Random Interleaver3 : commblkintrlv2/Random Interleaver  N=Len  seed=Seed
      settings: SourceProductBaseCode=CM
  Terminator1 : Terminator
  Terminator2 : Terminator
  Out1 : Outport
  wires:
  APP Decoder1/1 -> Random Deinterleaver/1
  APP Decoder/2 -> Terminator1/1
  APP Decoder1/2 -> Terminator2/1
  Random Deinterleaver/1 -> Delay/1, Hard Decision1/1(Lin)
  Random Interleaver3/1 -> APP Decoder1/1
  APP Decoder/1 -> Random Interleaver3/1
  Frame Reset/1 -> APP Decoder/1
  Delay/1 -> Frame Reset/1
  Discrete Pulse Generator/1 -> Frame Reset/2
  Hard Decision1/1(0/1) -> Out1/1
  In1/1 -> APP Decoder/2
  In2/1 -> APP Decoder1/2

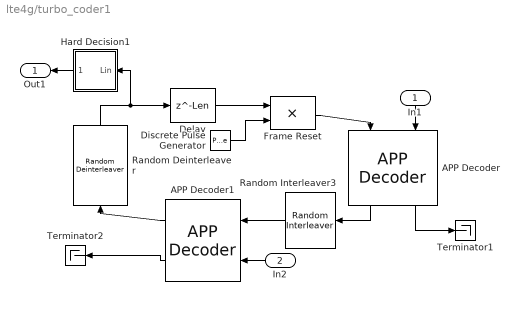
== system lte4g/turbo_coder1 ==
  In1 : Inport
  In2 : Inport  Port=2
  APP Decoder : commcnvcod2/APP Decoder  trellis=trellis  termMethod=Truncated  algorithm=Max*  maxStarNumScaleBits=3  disableLcOut=off
      settings: SourceProductBaseCode=CM
  APP Decoder1 : commcnvcod2/APP Decoder  trellis=trellis  termMethod=Truncated  algorithm=Max*  maxStarNumScaleBits=3  disableLcOut=off
      settings: SourceProductBaseCode=CM
  Delay : Delay  DelayLength=Len  InitialCondition=0  InputProcessing=Columns as channels (frame based)
  Discrete Pulse Generator : DiscretePulseGenerator  Period=Iter  PulseWidth=Iter-1  PhaseDelay=1
  Frame Reset : Product  InputSameDT=on  SaturateOnIntegerOverflow=on  OutDataTypeStr=Inherit: Same as first input
  Hard Decision1 : Subsystem  mask(Hard Decision){}
      mask help: Likelihood to binary transformation.
  Random Deinterleaver : commblkintrlv2/Random Deinterleaver  N=Len  seed=Seed
      settings: SourceProductBaseCode=CM
  Random Interleaver3 : commblkintrlv2/Random Interleaver  N=Len  seed=Seed
      settings: SourceProductBaseCode=CM
  Terminator1 : Terminator
  Terminator2 : Terminator
  Out1 : Outport
  wires:
  APP Decoder1/1 -> Random Deinterleaver/1
  APP Decoder/2 -> Terminator1/1
  APP Decoder1/2 -> Terminator2/1
  Random Deinterleaver/1 -> Delay/1, Hard Decision1/1(Lin)
  Random Interleaver3/1 -> APP Decoder1/1
  APP Decoder/1 -> Random Interleaver3/1
  Frame Reset/1 -> APP Decoder/1
  Delay/1 -> Frame Reset/1
  Discrete Pulse Generator/1 -> Frame Reset/2
  Hard Decision1/1(0/1) -> Out1/1
  In1/1 -> APP Decoder/2
  In2/1 -> APP Decoder1/2

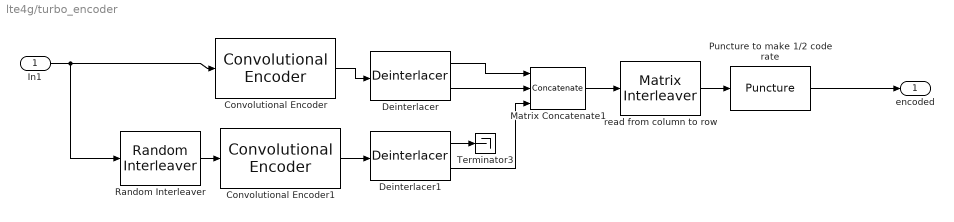
== system lte4g/turbo_encoder ==
  In1 : Inport
  Convolutional Encoder : commcnvcod2/Convolutional Encoder  trellis=trellis  opMode=Continuous  DelayedResetAction=off  hasIniStPort=off  hasFinStPort=off  usePuncVector=off  punctureVector=[ 1 1 0 1 0 1]'  reset=Unused parameter value
      settings: SourceProductBaseCode=CM
  Convolutional Encoder1 : commcnvcod2/Convolutional Encoder  trellis=trellis  opMode=Truncated (reset every frame)  DelayedResetAction=off  hasIniStPort=off  hasFinStPort=off  usePuncVector=off  punctureVector=[ 1 1 0 1 0 1]'  reset=Unused parameter value
      settings: SourceProductBaseCode=CM
  Deinterlacer : commsequence2/Deinterlacer
      settings: SourceProductBaseCode=CM
  Deinterlacer1 : commsequence2/Deinterlacer
      settings: SourceProductBaseCode=CM
  Matrix Concatenate1 : Concatenate  NumInputs=3  Mode=Multidimensional array
  Puncture to make 1/2 code rate : commsequence2/Puncture  punctureVector=[1 1 0 1 0 1].'
      settings: SourceProductBaseCode=CM
  Random Interleaver : commblkintrlv2/Random Interleaver  N=Len  seed=Seed
      settings: SourceProductBaseCode=CM
  Terminator3 : Terminator
  read from column to row : commblkintrlv2/Matrix Interleaver  Nrows=3  Ncols=Len
      settings: SourceProductBaseCode=CM
  encoded : Outport
  wires:
  In1/1 -> Convolutional Encoder/1, Random Interleaver/1
  Puncture to make 1/2 code rate/1 -> encoded/1
  Random Interleaver/1 -> Convolutional Encoder1/1
  Convolutional Encoder/1 -> Deinterlacer/1
  Convolutional Encoder1/1 -> Deinterlacer1/1
  Deinterlacer1/1 -> Terminator3/1
  Deinterlacer/1 -> Matrix Concatenate1/1
  Deinterlacer1/2 -> Matrix Concatenate1/3
  read from column to row/1 -> Puncture to make 1/2 code rate/1
  Matrix Concatenate1/1 -> read from column to row/1
  Deinterlacer/2 -> Matrix Concatenate1/2

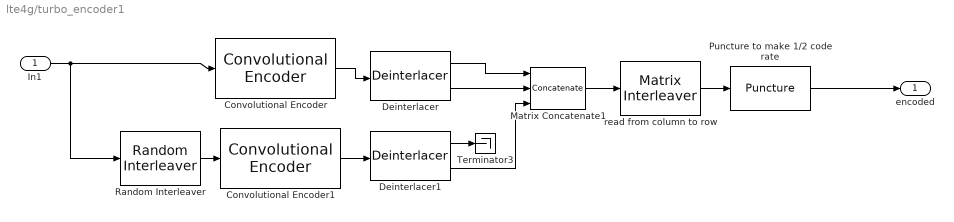
== system lte4g/turbo_encoder1 ==
  In1 : Inport
  Convolutional Encoder : commcnvcod2/Convolutional Encoder  trellis=trellis  opMode=Continuous  DelayedResetAction=off  hasIniStPort=off  hasFinStPort=off  usePuncVector=off  punctureVector=[ 1 1 0 1 0 1]'  reset=Unused parameter value
      settings: SourceProductBaseCode=CM
  Convolutional Encoder1 : commcnvcod2/Convolutional Encoder  trellis=trellis  opMode=Truncated (reset every frame)  DelayedResetAction=off  hasIniStPort=off  hasFinStPort=off  usePuncVector=off  punctureVector=[ 1 1 0 1 0 1]'  reset=Unused parameter value
      settings: SourceProductBaseCode=CM
  Deinterlacer : commsequence2/Deinterlacer
      settings: SourceProductBaseCode=CM
  Deinterlacer1 : commsequence2/Deinterlacer
      settings: SourceProductBaseCode=CM
  Matrix Concatenate1 : Concatenate  NumInputs=3  Mode=Multidimensional array
  Puncture to make 1/2 code rate : commsequence2/Puncture  punctureVector=[1 1 0 1 0 1].'
      settings: SourceProductBaseCode=CM
  Random Interleaver : commblkintrlv2/Random Interleaver  N=Len  seed=Seed
      settings: SourceProductBaseCode=CM
  Terminator3 : Terminator
  read from column to row : commblkintrlv2/Matrix Interleaver  Nrows=3  Ncols=Len
      settings: SourceProductBaseCode=CM
  encoded : Outport
  wires:
  In1/1 -> Convolutional Encoder/1, Random Interleaver/1
  Puncture to make 1/2 code rate/1 -> encoded/1
  Random Interleaver/1 -> Convolutional Encoder1/1
  Convolutional Encoder/1 -> Deinterlacer/1
  Convolutional Encoder1/1 -> Deinterlacer1/1
  Deinterlacer1/1 -> Terminator3/1
  Deinterlacer/1 -> Matrix Concatenate1/1
  Deinterlacer1/2 -> Matrix Concatenate1/3
  read from column to row/1 -> Puncture to make 1/2 code rate/1
  Matrix Concatenate1/1 -> read from column to row/1
  Deinterlacer/2 -> Matrix Concatenate1/2

== system lte4g/Subsystem/Subsystem ==
  In1 : Inport
  Selector3 : Selector  NumberOfDimensions=2  InputPortWidth=64  IndexOptions=Index vector (dialog),Select all  Indices=[39:64,1:64],-1  OutputSizes=1
  Out1 : Outport
  wires:
  Selector3/1 -> Out1/1
  In1/1 -> Selector3/1

== system lte4g/Subsystem/Subsystem1 ==
  In1 : Inport
  Selector : Selector  NumberOfDimensions=2  InputPortWidth=64  IndexOptions=Index vector (dialog),Select all  Indices=[12:64,1:11],-1  OutputSizes=1
  Zero Pad : dspsigops/Pad  padAlong=Columns and rows  dimsToPad=1  valSrc=Specify via dialog  padVal=0  spec=Output size  padNumOutRowsSpecMethod=User-specified  numOutRows=64  padNumOutColsSpecMethod=User-specified  numOutCols=2  isVarDimsMode=off  padBeginning=0  padEnd=0  outSizeMode=User-specified  outSize=1  padSigAt=End  trunc_flag=None  roundingMode=Floor  overflowMode=off  truncOrWrapMode=Truncate  wrap_flag=None
      settings: SourceProductBaseCode=DS
  Out1 : Outport
  wires:
  Zero Pad/1 -> Selector/1
  In1/1 -> Zero Pad/1
  Selector/1 -> Out1/1

== system lte4g/Subsystem1/Subsystem ==
  In1 : Inport
  Selector4 : Selector  NumberOfDimensions=2  InputPortWidth=78  IndexOptions=Index vector (dialog),Select all  Indices=[27:90],-1  OutputSizes=1
  Out1 : Outport
  wires:
  Selector4/1 -> Out1/1
  In1/1 -> Selector4/1

== system lte4g/Subsystem17/Subsystem ==
  In1 : Inport
  Enable : EnablePort
  Math Function : Math  Operator=reciprocal  SignedPower=on  SaturateOnIntegerOverflow=on
  Out1 : Outport
  wires:
  In1/1 -> Math Function/1
  Math Function/1 -> Out1/1

== system lte4g/Subsystem17/Subsystem4 ==
  Enable : EnablePort
  Frame Status Conversion2 : dspobslib/Frame Status Conversion  growRefPort=off  outframe=Frame-based
      settings: SourceProductBaseCode=DS
  Math Function : Math  Operator=reciprocal  SignedPower=on  SaturateOnIntegerOverflow=on
  PN Sequence Generator : commseqgen3/PN Sequence Generator  poly=[1 0 0 0 0 1 1]  ini_sta=[0 0 0 0 0 1]  outBitMaskSource=Dialog parameter  shift=0  outVarSiz=off  maxOutSizeMode=Dialog parameter  maxOutSize=[10 1]  Ts=16e-5/2/23  sampPerFrame=23  reset=off  bitPackedOutputs=off  outDataType=double  numPackedBits=8  bitPackDataSigned=off  bitPackedOutDType=double
  Unipolar to Bipolar Converter : commutil2/Unipolar to Bipolar Converter  M=2  polarity=Positive  dataType=Inherit via internal rule
  Out1 : Outport
  wires:
  PN Sequence Generator/1 -> Unipolar to Bipolar Converter/1
  Frame Status Conversion2/1 -> Out1/1
  Math Function/1 -> Frame Status Conversion2/1
  Unipolar to Bipolar Converter/1 -> Math Function/1

== system lte4g/Subsystem5/Subsystem ==
  In1 : Inport
  Enable : EnablePort
  Math Function : Math  Operator=reciprocal  SignedPower=on  SaturateOnIntegerOverflow=on
  Out1 : Outport
  wires:
  In1/1 -> Math Function/1
  Math Function/1 -> Out1/1

== system lte4g/Subsystem5/Subsystem4 ==
  Enable : EnablePort
  Frame Status Conversion2 : dspobslib/Frame Status Conversion  growRefPort=off  outframe=Frame-based
      settings: SourceProductBaseCode=DS
  Math Function : Math  Operator=reciprocal  SignedPower=on  SaturateOnIntegerOverflow=on
  PN Sequence Generator : commseqgen3/PN Sequence Generator  poly=[1 0 0 0 0 1 1]  ini_sta=[0 0 0 0 0 1]  outBitMaskSource=Dialog parameter  shift=0  outVarSiz=off  maxOutSizeMode=Dialog parameter  maxOutSize=[10 1]  Ts=16e-5/2/23  sampPerFrame=23  reset=off  bitPackedOutputs=off  outDataType=double  numPackedBits=8  bitPackDataSigned=off  bitPackedOutDType=double
  Unipolar to Bipolar Converter : commutil2/Unipolar to Bipolar Converter  M=2  polarity=Positive  dataType=Inherit via internal rule
  Out1 : Outport
  wires:
  PN Sequence Generator/1 -> Unipolar to Bipolar Converter/1
  Frame Status Conversion2/1 -> Out1/1
  Math Function/1 -> Frame Status Conversion2/1
  Unipolar to Bipolar Converter/1 -> Math Function/1

== system lte4g/Subsystem8/Subsystem ==
  In1 : Inport
  Selector3 : Selector  NumberOfDimensions=2  InputPortWidth=64  IndexOptions=Index vector (dialog),Select all  Indices=[39:64,1:64],-1  OutputSizes=1
  Out1 : Outport
  wires:
  Selector3/1 -> Out1/1
  In1/1 -> Selector3/1

== system lte4g/Subsystem8/Subsystem1 ==
  In1 : Inport
  Selector : Selector  NumberOfDimensions=2  InputPortWidth=64  IndexOptions=Index vector (dialog),Select all  Indices=[12:64,1:11],-1  OutputSizes=1
  Zero Pad : dspsigops/Pad  padAlong=Columns and rows  dimsToPad=1  valSrc=Specify via dialog  padVal=0  spec=Output size  padNumOutRowsSpecMethod=User-specified  numOutRows=64  padNumOutColsSpecMethod=User-specified  numOutCols=2  isVarDimsMode=off  padBeginning=0  padEnd=0  outSizeMode=User-specified  outSize=1  padSigAt=End  trunc_flag=None  roundingMode=Floor  overflowMode=off  truncOrWrapMode=Truncate  wrap_flag=None
      settings: SourceProductBaseCode=DS
  Out1 : Outport
  wires:
  Zero Pad/1 -> Selector/1
  In1/1 -> Zero Pad/1
  Selector/1 -> Out1/1

== system lte4g/Subsystem9/Subsystem ==
  In1 : Inport
  Selector4 : Selector  NumberOfDimensions=2  InputPortWidth=78  IndexOptions=Index vector (dialog),Select all  Indices=[27:90],-1  OutputSizes=1
  Out1 : Outport
  wires:
  Selector4/1 -> Out1/1
  In1/1 -> Selector4/1

== system lte4g/turbo_coder/Hard Decision1 ==
  Lin : Inport
  Constant : Constant  Value=0
  Relational Operator : RelationalOperator  RndMeth=Nearest  InputSameDT=on
  0/1 : Outport
  wires:
  Constant/1 -> Relational Operator/2
  Lin/1 -> Relational Operator/1
  Relational Operator/1 -> 0/1/1

== system lte4g/turbo_coder1/Hard Decision1 ==
  Lin : Inport
  Constant : Constant  Value=0
  Relational Operator : RelationalOperator  RndMeth=Nearest  InputSameDT=on
  0/1 : Outport
  wires:
  Constant/1 -> Relational Operator/2
  Lin/1 -> Relational Operator/1
  Relational Operator/1 -> 0/1/1

== matlab function lte4g/Embedded MATLAB Function ==
  data: s2 input; ber output; s8 input
function ber = fcn(s2,s8)
y=s2-s8;
z=0;
for i=1:20
    if y(i)~=0
        z=z+1;
    end
    
end
ber=z/(length(s2)*38);

== matlab function lte4g/Embedded MATLAB Function2 ==
  data: s8 input; cer output
function cer = fcn(s8)
c1 = s8';
c=0;
for i=1:length(c1)
    c= c+ (c1(i)*2^(length(c1)-i));
end 
cer = c;

== matlab function lte4g/MATLAB Function ==
  data: u input; y output
function y = fcn(u)
    if u>= 0.05
        y=1;  
        
    else 
        y=0;
%          pause(10.0);
    end
end

== matlab function lte4g/Embedded MATLAB Function3 ==
  data: s2 input; ber output
function ber = fcn(s2)
%x = de2bi(s2)
%y = len(x)
b = zeros(20,1);
a = (de2bi(s2))';
la = length(a);
lb = length(b);
for i = 1:la
    b(lb+1-i) = a(i);  
end

ber = b;

== matlab function lte4g/Embedded MATLAB Function4 ==
  data: s2 input; ber output; s8 input
function ber = fcn(s2,s8)
y=s2-s8;
z=0;
for i=1:20
    if y(i)~=0
        z=z+1;
    end
    
end
ber=z/(length(s2)*38);

== matlab function lte4g/Embedded MATLAB Function5 ==
  data: s8 input; cer output
function cer = fcn(s8)
c1 = s8';
c=0;
for i=1:length(c1)
    c= c+ (c1(i)*2^(length(c1)-i));
end 
cer = c;

== matlab function lte4g/Embedded MATLAB Function6 ==
  data: s8 input; cer output
function cer = fcn(s8)
if s8>1.03
    c= 1.03;
else
    c=s8;
end
cer = c;

== matlab function lte4g/Embedded MATLAB Function1 ==
  data: s2 input; ber output
function ber = fcn(s2)
%x = de2bi(s2)
%y = len(x)
b = zeros(20,1);
a = (de2bi(s2))';
la = length(a);
lb = length(b);
for i = 1:la
    b(lb+1-i) = a(i);  
end

ber = b;
